simulink library "FunctionCallDivider"  (R2019b)
settings: Solver=VariableStepAuto  StartTime=0.0  StopTime=10.0  RelTol=1e-3
libraries: simulink x1
settings Model: Creator=Nick  LastModifiedBy=Nick
settings DataIOCC: ReturnWorkspaceOutputs=off
settings DebuggingCC: ArithmeticOperatorsInVariantConditions=warning
settings SFSimCC: CustomCodeUndefinedFunction=UseInterfaceOnly

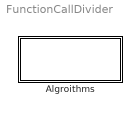
== system FunctionCallDivider ==
  Algroithms : Subsystem

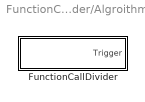
== system FunctionCallDivider/Algroithms ==
  FunctionCallDivider : Subsystem  mask{counts=100}
      mask prompts: counts "Count"
      mask Display:
      | color('blue');
      | disp(sprintf(['Function Call Divider\n', num2str(counts), 'x\n']));

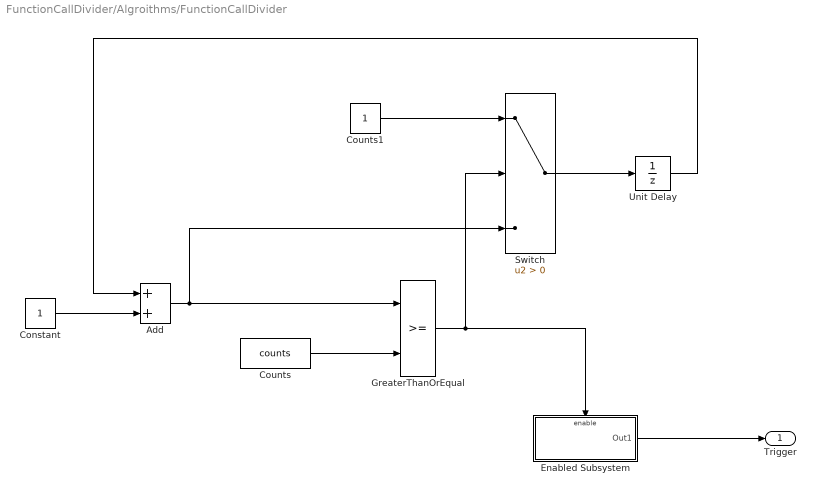
== system FunctionCallDivider/Algroithms/FunctionCallDivider ==
  Add : Sum
  Constant : Constant
  Counts : Constant  Value=counts
  Counts1 : Constant
  Enabled Subsystem : Subsystem  TreatAsAtomicUnit=on
  GreaterThanOrEqual : RelationalOperator  OutDataTypeStr=boolean  RndMeth=Simplest
  Switch : Switch  Criteria=u2 > Threshold
  Unit Delay : UnitDelay  SampleTime=-1  HasFrameUpgradeWarning=on
  Trigger : Outport
  wires:
  Constant/1 -> Add/2
  Add/1 -> Switch/3, GreaterThanOrEqual/1
  GreaterThanOrEqual/1 -> Switch/2, Enabled Subsystem/Enable
  Enabled Subsystem/1(Out1) -> Trigger/1
  Counts/1 -> GreaterThanOrEqual/2
  Unit Delay/1 -> Add/1
  Counts1/1 -> Switch/1
  Switch/1 -> Unit Delay/1

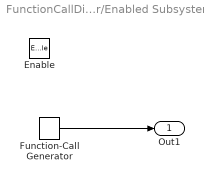
== system FunctionCallDivider/Algroithms/FunctionCallDivider/Enabled Subsystem ==
  Enable : EnablePort
  Function-Call Generator : simulink/Ports & Subsystems/Function-Call Generator  sample_time=-1  numberOfIterations=1
  Out1 : Outport
  wires:
  Function-Call Generator/1 -> Out1/1
